simulink model "AdaptiveSync_2_3"  (R2016a)
settings: Solver=ode23tb  SolverMode=SingleTasking  StartTime=0.0  StopTime=80  RelTol=1e-3
values from neighbouring files (symbols this model uses):
  A1 = [0,1;-2,-1]    [Adaptive_Synchronization.m]
  A2 = [0,1;-2.5,-0.75]    [Adaptive_Synchronization.m]
  A3 = [0,1;-2,-1.25]    [Adaptive_Synchronization.m]
  A4 = [0,1;-1,-0.5]    [Adaptive_Synchronization.m]
  A5 = [0,1;-1,-0.75]    [Adaptive_Synchronization.m]
  Aer = kron(L,eye(2))    [Adaptive_Synchronization.m]
  Am = [0 1;-(0.7)^2, 0]    [Adaptive_Synchronization.m]
  B1 = [0;1]    [Adaptive_Synchronization.m]
  B2 = [0;1]    [Adaptive_Synchronization.m]
  B3 = [0;1]    [Adaptive_Synchronization.m]
  B4 = [0;1]    [Adaptive_Synchronization.m]
  B5 = [0;1]    [Adaptive_Synchronization.m]
  Bm = [0;1]    [Adaptive_Synchronization.m]
  Cm = eye(2)    [Adaptive_Synchronization.m]
  Dm = [0;0]    [Adaptive_Synchronization.m]
  Fadapt = [-15 -25]    [Adaptive_Synchronization.m]
  gamma = [50 50;50 50; 50 50; 50 50; 100 100]'    [Adaptive_Synchronization.m]
  P = care(Am+lambda(2)*Bm*Fadapt,[0;0],-Q)    [Adaptive_Synchronization.m]
  x01 = [-0.5;1]    [Adaptive_Synchronization.m]
  x02 = [0.5;-1]    [Adaptive_Synchronization.m]
  x03 = [1;0.5]    [Adaptive_Synchronization.m]
  x04 = [-1;-0.5]    [Adaptive_Synchronization.m]
  x05 = [0;0]    [Adaptive_Synchronization.m]
  x0m = [0;1]    [Adaptive_Synchronization.m]
settings Model: Creator=tdvos  LastModifiedBy=danielvos
settings SolverCC: ZeroCrossAlgorithm=Adaptive
settings DebuggingCC: SFUnexpectedBacktrackingDiag=error  SFNoUnconditionalDefaultTransitionDiag=error
settings GRTTargetCC: TargetLangStandard=C99 (ISO)  GeneratePreprocessorConditionals=Use local settings
settings ConfigComp: CovMetricSettings=dwe  CovHtmlReporting=off  CovSaveCumulativeToWorkspaceVar=off  CovSaveSingleToWorkspaceVar=off  CovExternalEMLEnable=on

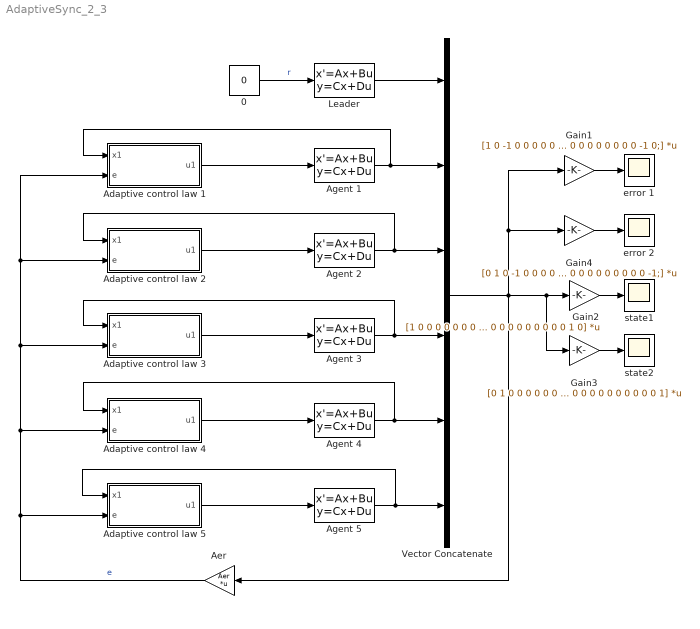
== system AdaptiveSync_2_3 ==
  0 : Constant  Value=0
  Adaptive control law 1 : Subsystem
  Adaptive control law 2 : Subsystem
  Adaptive control law 3 : Subsystem
  Adaptive control law 4 : Subsystem
  Adaptive control law 5 : Subsystem
  Aer : Gain  Gain=Aer  Multiplication=Matrix(K*u)
  Agent 1 : StateSpace  A=A1  B=B1  C=eye(2)  D=zeros(2,1)  X0=x01
  Agent 2 : StateSpace  A=A2  B=B2  C=eye(2)  D=zeros(2,1)  X0=x02
  Agent 3 : StateSpace  A=A3  B=B3  C=eye(2)  D=zeros(2,1)  X0=x03
  Agent 4 : StateSpace  A=A4  B=B4  C=eye(2)  D=zeros(2,1)  X0=x04
  Agent 5 : StateSpace  A=A5  B=B5  C=eye(2)  D=zeros(2,1)  X0=x05
  Gain1 : Gain  Gain=[1 0 -1 0 0 0 0 0 0 0 0 0;1 0 0 0 -1 0 0 0 0 0 0 0;1 0 0 0 0 0 -1 0 0 0 0 0;1 0 0 0 0 0 0 0 -1 0 0 0;1 0 0 0 0 0 0 0 0 0 -1 0;]  Multiplication=Matrix(K*u)
  Gain2 : Gain  Gain=[1 0 0 0 0 0 0 0 0 0 0 0;0 0 1 0 0 0 0 0 0 0 0 0;0 0 0 0 1 0 0 0 0 0 0 0;0 0 0 0 0 0 1 0 0 0 0 0;0 0 0 0 0 0 0 0 1 0 0 0;0 0 0 0 0 0 0 0 0 0 1 0]  Multiplication=Matrix(K*u)
  Gain3 : Gain  Gain=[0 1 0 0 0 0 0 0 0 0 0 0;0 0 0 1 0 0 0 0 0 0 0 0;0 0 0 0 0 1 0 0 0 0 0 0;0 0 0 0 0 0 0 1 0 0 0 0;0 0 0 0 0 0 0 0 0 1 0 0; 0 0 0 0 0 0 0 0 0 0 0 1]  Multiplication=Matrix(K*u)
  Gain4 : Gain  Gain=[0 1 0 -1 0 0 0 0 0 0 0 0;0 1 0 0 0 -1 0 0 0 0 0 0;0 1 0 0 0 0 0 -1 0 0 0 0;0 1 0 0 0 0 0 0 0 -1 0 0;0 1 0 0 0 0 0 0 0 0 0 -1;]  Multiplication=Matrix(K*u)
  Leader : StateSpace  A=Am  B=Bm  C=Cm  D=Dm  X0=x0m
  Vector Concatenate : Concatenate  NumInputs=6
  error 1 : Scope
  error 2 : Scope
  state1 : Scope
  state2 : Scope
  wires:
  Agent 1/1 -> Adaptive control law 1/1(x1), Vector Concatenate/2
  Agent 2/1 -> Adaptive control law 2/1(x1), Vector Concatenate/3
  Agent 3/1 -> Adaptive control law 3/1(x1), Vector Concatenate/4
  Agent 4/1 -> Vector Concatenate/5, Adaptive control law 4/1(x1)
  Agent 5/1 -> Adaptive control law 5/1(x1), Vector Concatenate/6
  Aer/1 -> Adaptive control law 5/2(e), Adaptive control law 4/2(e), Adaptive control law 2/2(e), Adaptive control law 1/2(e), Adaptive control law 3/2(e)  "e"
  Adaptive control law 1/1(u1) -> Agent 1/1
  0/1 -> Leader/1  "r"
  Leader/1 -> Vector Concatenate/1
  Adaptive control law 2/1(u1) -> Agent 2/1
  Adaptive control law 3/1(u1) -> Agent 3/1
  Adaptive control law 4/1(u1) -> Agent 4/1
  Adaptive control law 5/1(u1) -> Agent 5/1
  Gain3/1 -> state2/1
  Vector Concatenate/1 -> Gain4/1, Gain1/1, Gain3/1, Gain2/1, Aer/1
  Gain2/1 -> state1/1
  Gain1/1 -> error 1/1
  Gain4/1 -> error 2/1

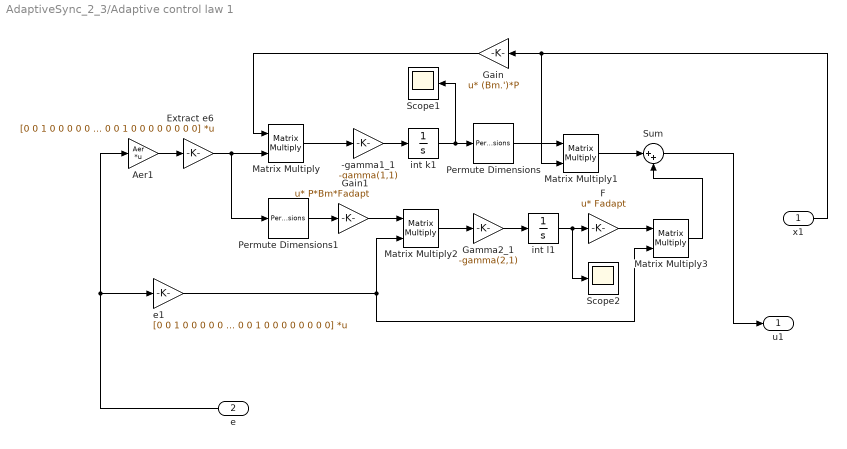
== system AdaptiveSync_2_3/Adaptive control law 1 ==
  x1 : Inport
  e : Inport  Port=2
  -gamma1_1 : Gain  Gain=-gamma(1,1)
  Aer1 : Gain  Gain=Aer  Multiplication=Matrix(K*u)
  Extract e6 : Gain  Gain=[0 0 1 0 0 0 0 0 0 0 0 0; 0 0 0 1 0 0 0 0 0 0 0 0]  Multiplication=Matrix(K*u)
  F : Gain  Gain=Fadapt  Multiplication=Matrix(u*K)
  Gain : Gain  Gain=(Bm.')*P  Multiplication=Matrix(u*K)
  Gain1 : Gain  Gain=P*Bm*Fadapt  Multiplication=Matrix(u*K)
  "Gamma2_1 " : Gain  Gain=-gamma(2,1)
  Matrix Multiply{,1..3} (4 alike) : Product  Multiplication=Matrix(*)
  Permute Dimensions : PermuteDimensions
  Permute Dimensions1 : PermuteDimensions
  Scope1 : Scope
  Scope2 : Scope
  Sum : Sum  Inputs=|++
  e1 : Gain  Gain=[0 0 1 0 0 0 0 0 0 0 0 0; 0 0 0 1 0 0 0 0 0 0 0 0]  Multiplication=Matrix(K*u)
  int k1 : Integrator  InitialCondition=[0;0]
  int l1 : Integrator
  u1 : Outport
  wires:
  Sum/1 -> u1/1
  Matrix Multiply3/1 -> Sum/2
  F/1 -> Matrix Multiply3/1
  Matrix Multiply/1 -> -gamma1_1/1
  -gamma1_1/1 -> int k1/1
  Permute Dimensions/1 -> Matrix Multiply1/1
  Matrix Multiply2/1 -> "Gamma2_1 "/1
  e/1 -> Aer1/1, e1/1
  Gain1/1 -> Matrix Multiply2/1
  Gain/1 -> Matrix Multiply/1
  Aer1/1 -> Extract e6/1
  "Gamma2_1 "/1 -> int l1/1
  Extract e6/1 -> Permute Dimensions1/1, Matrix Multiply/2
  e1/1 -> Matrix Multiply2/2, Matrix Multiply3/2
  Matrix Multiply1/1 -> Sum/1
  int l1/1 -> Scope2/1, F/1
  Permute Dimensions1/1 -> Gain1/1
  x1/1 -> Matrix Multiply1/2, Gain/1
  int k1/1 -> Scope1/1, Permute Dimensions/1

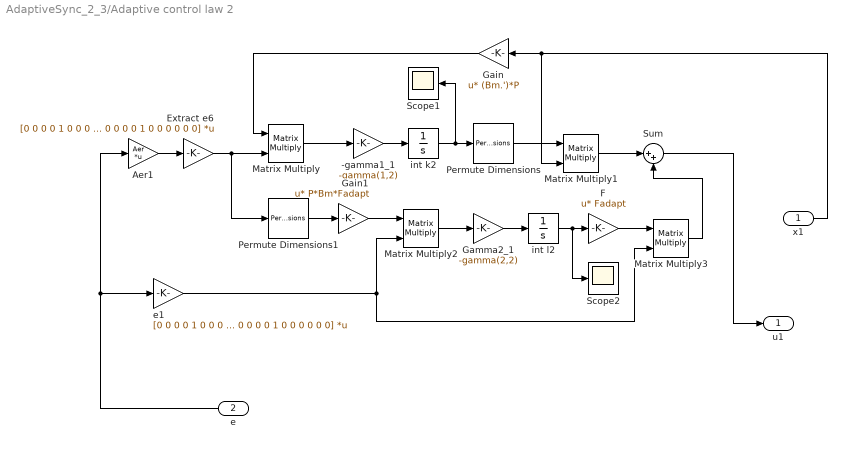
== system AdaptiveSync_2_3/Adaptive control law 2 ==
  x1 : Inport
  e : Inport  Port=2
  -gamma1_1 : Gain  Gain=-gamma(1,2)
  Aer1 : Gain  Gain=Aer  Multiplication=Matrix(K*u)
  Extract e6 : Gain  Gain=[0 0 0 0 1 0 0 0 0 0 0 0; 0 0 0 0 0 1 0 0 0 0 0 0]  Multiplication=Matrix(K*u)
  F : Gain  Gain=Fadapt  Multiplication=Matrix(u*K)
  Gain : Gain  Gain=(Bm.')*P  Multiplication=Matrix(u*K)
  Gain1 : Gain  Gain=P*Bm*Fadapt  Multiplication=Matrix(u*K)
  "Gamma2_1 " : Gain  Gain=-gamma(2,2)
  Matrix Multiply{,1..3} (4 alike) : Product  Multiplication=Matrix(*)
  Permute Dimensions : PermuteDimensions
  Permute Dimensions1 : PermuteDimensions
  Scope1 : Scope
  Scope2 : Scope
  Sum : Sum  Inputs=|++
  e1 : Gain  Gain=[0 0 0 0 1 0 0 0 0 0 0 0; 0 0 0 0 0 1 0 0 0 0 0 0]  Multiplication=Matrix(K*u)
  int k2 : Integrator  InitialCondition=[0;0]
  int l2 : Integrator
  u1 : Outport
  wires:
  Sum/1 -> u1/1
  Matrix Multiply3/1 -> Sum/2
  F/1 -> Matrix Multiply3/1
  Matrix Multiply/1 -> -gamma1_1/1
  -gamma1_1/1 -> int k2/1
  Permute Dimensions/1 -> Matrix Multiply1/1
  Matrix Multiply2/1 -> "Gamma2_1 "/1
  e/1 -> Aer1/1, e1/1
  Gain1/1 -> Matrix Multiply2/1
  Gain/1 -> Matrix Multiply/1
  Aer1/1 -> Extract e6/1
  "Gamma2_1 "/1 -> int l2/1
  Extract e6/1 -> Permute Dimensions1/1, Matrix Multiply/2
  e1/1 -> Matrix Multiply2/2, Matrix Multiply3/2
  Matrix Multiply1/1 -> Sum/1
  int l2/1 -> Scope2/1, F/1
  Permute Dimensions1/1 -> Gain1/1
  x1/1 -> Matrix Multiply1/2, Gain/1
  int k2/1 -> Scope1/1, Permute Dimensions/1

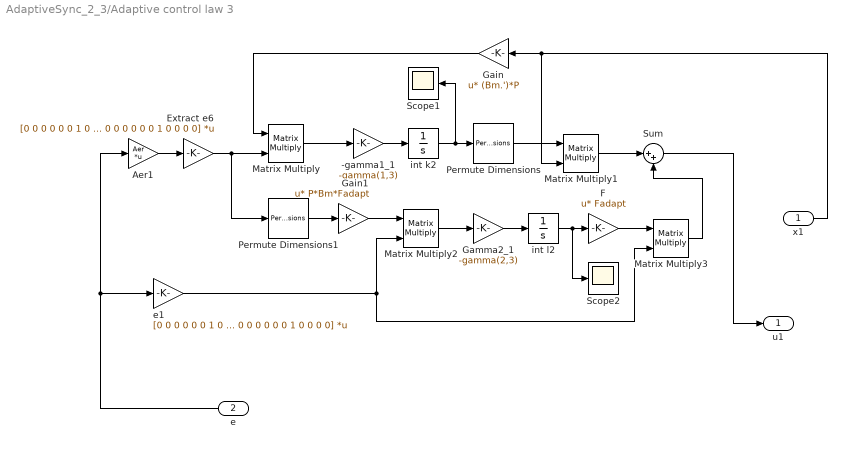
== system AdaptiveSync_2_3/Adaptive control law 3 ==
  x1 : Inport
  e : Inport  Port=2
  -gamma1_1 : Gain  Gain=-gamma(1,3)
  Aer1 : Gain  Gain=Aer  Multiplication=Matrix(K*u)
  Extract e6 : Gain  Gain=[0 0 0 0 0 0 1 0 0 0 0 0; 0 0 0 0 0 0 0 1 0 0 0 0]  Multiplication=Matrix(K*u)
  F : Gain  Gain=Fadapt  Multiplication=Matrix(u*K)
  Gain : Gain  Gain=(Bm.')*P  Multiplication=Matrix(u*K)
  Gain1 : Gain  Gain=P*Bm*Fadapt  Multiplication=Matrix(u*K)
  "Gamma2_1 " : Gain  Gain=-gamma(2,3)
  Matrix Multiply{,1..3} (4 alike) : Product  Multiplication=Matrix(*)
  Permute Dimensions : PermuteDimensions
  Permute Dimensions1 : PermuteDimensions
  Scope1 : Scope
  Scope2 : Scope
  Sum : Sum  Inputs=|++
  e1 : Gain  Gain=[0 0 0 0 0 0 1 0 0 0 0 0; 0 0 0 0 0 0 0 1 0 0 0 0]  Multiplication=Matrix(K*u)
  int k2 : Integrator  InitialCondition=[0;0]
  int l2 : Integrator
  u1 : Outport
  wires:
  Sum/1 -> u1/1
  Matrix Multiply3/1 -> Sum/2
  F/1 -> Matrix Multiply3/1
  Matrix Multiply/1 -> -gamma1_1/1
  -gamma1_1/1 -> int k2/1
  Permute Dimensions/1 -> Matrix Multiply1/1
  Matrix Multiply2/1 -> "Gamma2_1 "/1
  e/1 -> Aer1/1, e1/1
  Gain1/1 -> Matrix Multiply2/1
  Gain/1 -> Matrix Multiply/1
  Aer1/1 -> Extract e6/1
  "Gamma2_1 "/1 -> int l2/1
  Extract e6/1 -> Permute Dimensions1/1, Matrix Multiply/2
  e1/1 -> Matrix Multiply2/2, Matrix Multiply3/2
  Matrix Multiply1/1 -> Sum/1
  int l2/1 -> Scope2/1, F/1
  Permute Dimensions1/1 -> Gain1/1
  x1/1 -> Matrix Multiply1/2, Gain/1
  int k2/1 -> Scope1/1, Permute Dimensions/1

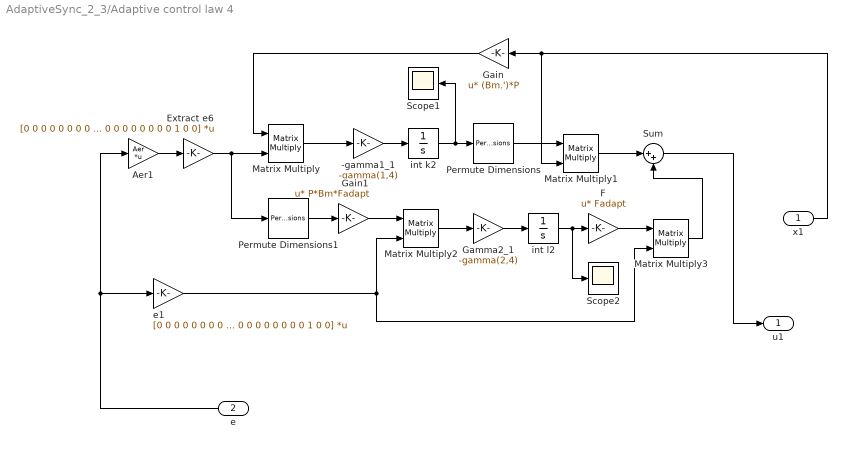
== system AdaptiveSync_2_3/Adaptive control law 4 ==
  x1 : Inport
  e : Inport  Port=2
  -gamma1_1 : Gain  Gain=-gamma(1,4)
  Aer1 : Gain  Gain=Aer  Multiplication=Matrix(K*u)
  Extract e6 : Gain  Gain=[0 0 0 0 0 0 0 0 1 0 0 0; 0 0 0 0 0 0 0 0 0 1 0 0]  Multiplication=Matrix(K*u)
  F : Gain  Gain=Fadapt  Multiplication=Matrix(u*K)
  Gain : Gain  Gain=(Bm.')*P  Multiplication=Matrix(u*K)
  Gain1 : Gain  Gain=P*Bm*Fadapt  Multiplication=Matrix(u*K)
  "Gamma2_1 " : Gain  Gain=-gamma(2,4)
  Matrix Multiply{,1..3} (4 alike) : Product  Multiplication=Matrix(*)
  Permute Dimensions : PermuteDimensions
  Permute Dimensions1 : PermuteDimensions
  Scope1 : Scope
  Scope2 : Scope
  Sum : Sum  Inputs=|++
  e1 : Gain  Gain=[0 0 0 0 0 0 0 0 1 0 0 0; 0 0 0 0 0 0 0 0 0 1 0 0]  Multiplication=Matrix(K*u)
  int k2 : Integrator  InitialCondition=[0;0]
  int l2 : Integrator
  u1 : Outport
  wires:
  Sum/1 -> u1/1
  Matrix Multiply3/1 -> Sum/2
  F/1 -> Matrix Multiply3/1
  Matrix Multiply/1 -> -gamma1_1/1
  -gamma1_1/1 -> int k2/1
  Permute Dimensions/1 -> Matrix Multiply1/1
  Matrix Multiply2/1 -> "Gamma2_1 "/1
  e/1 -> Aer1/1, e1/1
  Gain1/1 -> Matrix Multiply2/1
  Gain/1 -> Matrix Multiply/1
  Aer1/1 -> Extract e6/1
  "Gamma2_1 "/1 -> int l2/1
  Extract e6/1 -> Permute Dimensions1/1, Matrix Multiply/2
  e1/1 -> Matrix Multiply2/2, Matrix Multiply3/2
  Matrix Multiply1/1 -> Sum/1
  int l2/1 -> Scope2/1, F/1
  Permute Dimensions1/1 -> Gain1/1
  x1/1 -> Matrix Multiply1/2, Gain/1
  int k2/1 -> Scope1/1, Permute Dimensions/1

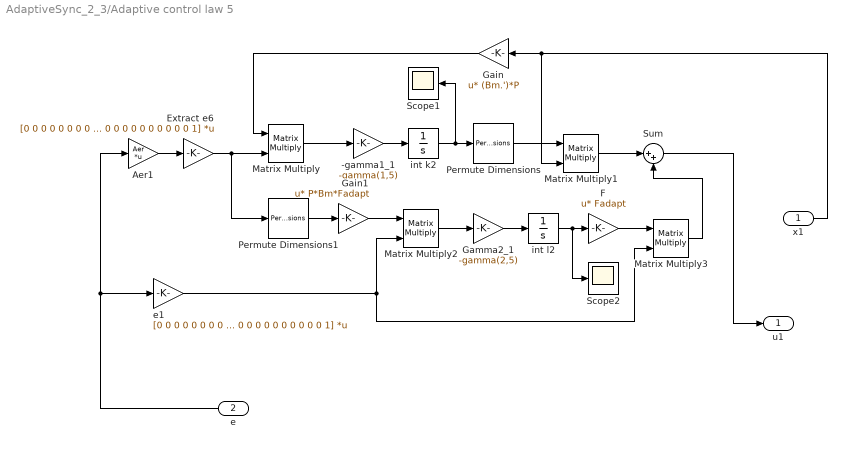
== system AdaptiveSync_2_3/Adaptive control law 5 ==
  x1 : Inport
  e : Inport  Port=2
  -gamma1_1 : Gain  Gain=-gamma(1,5)
  Aer1 : Gain  Gain=Aer  Multiplication=Matrix(K*u)
  Extract e6 : Gain  Gain=[0 0 0 0 0 0 0 0 0 0 1 0; 0 0 0 0 0 0 0 0 0 0 0 1]  Multiplication=Matrix(K*u)
  F : Gain  Gain=Fadapt  Multiplication=Matrix(u*K)
  Gain : Gain  Gain=(Bm.')*P  Multiplication=Matrix(u*K)
  Gain1 : Gain  Gain=P*Bm*Fadapt  Multiplication=Matrix(u*K)
  "Gamma2_1 " : Gain  Gain=-gamma(2,5)
  Matrix Multiply{,1..3} (4 alike) : Product  Multiplication=Matrix(*)
  Permute Dimensions : PermuteDimensions
  Permute Dimensions1 : PermuteDimensions
  Scope1 : Scope
  Scope2 : Scope
  Sum : Sum  Inputs=|++
  e1 : Gain  Gain=[0 0 0 0 0 0 0 0 0 0 1 0; 0 0 0 0 0 0 0 0 0 0 0 1]  Multiplication=Matrix(K*u)
  int k2 : Integrator  InitialCondition=[0;0]
  int l2 : Integrator
  u1 : Outport
  wires:
  Sum/1 -> u1/1
  Matrix Multiply3/1 -> Sum/2
  F/1 -> Matrix Multiply3/1
  Matrix Multiply/1 -> -gamma1_1/1
  -gamma1_1/1 -> int k2/1
  Permute Dimensions/1 -> Matrix Multiply1/1
  Matrix Multiply2/1 -> "Gamma2_1 "/1
  e/1 -> Aer1/1, e1/1
  Gain1/1 -> Matrix Multiply2/1
  Gain/1 -> Matrix Multiply/1
  Aer1/1 -> Extract e6/1
  "Gamma2_1 "/1 -> int l2/1
  Extract e6/1 -> Permute Dimensions1/1, Matrix Multiply/2
  e1/1 -> Matrix Multiply2/2, Matrix Multiply3/2
  Matrix Multiply1/1 -> Sum/1
  int l2/1 -> Scope2/1, F/1
  Permute Dimensions1/1 -> Gain1/1
  x1/1 -> Matrix Multiply1/2, Gain/1
  int k2/1 -> Scope1/1, Permute Dimensions/1
